simulink model "Automotive_Wiper"  (R2022b)
settings: Solver=FixedStepAuto  StartTime=0.0  StopTime=16  FixedStep=0.01  RelTol=1e-3
model workspace (MAT data in the model file):
  lowPathFilterGain = Simulink.Parameter
  lowPathFilterGain.Value = 0.1
  lowPathFilterGain.DataType = 'double'
  lowPathFilterGain.Complexity = 'real'
  lowPathFilterGain.Dimensions = [1 1]
undefined symbols (not defined in the file or in its folder): sigbuilder_block
libraries: simulink x1
settings Model: NumberOfSteps=100  VariantFading=off  Creator=mohsa  LastModifiedBy=mohsa
settings OptimizationCC: DefaultParameterBehavior=Inlined  UseDivisionForNetSlopeComputation=on  GainParamInheritBuiltInType=on  UseFloatMulNetSlope=on  InlineInvariantSignals=on  PassReuseOutputArgsAs=Individual arguments  ZeroExternalMemoryAtStartup=off  ZeroInternalMemoryAtStartup=off  NoFixptDivByZeroProtection=on  EfficientFloat2IntCast=on  LifeSpan=1  OptimizeBlockOrder=speed  DifferentSizesBufferReuse=on  EfficientTunableParamExpr=on
settings DebuggingCC: ParameterPrecisionLossMsg=none  ParameterTunabilityLossMsg=error
settings HardwareCC: ProdBitPerPointer=32  ProdBitPerSizeT=32  ProdBitPerPtrDiffT=32  ProdLargestAtomicInteger=Long  ProdLargestAtomicFloat=Double  ProdWordSize=32  ProdLongLongMode=on  ProdHWDeviceType=ARM Compatible->ARM Cortex-M
settings SFSimCC: MATLABDynamicMemAlloc=off
settings RTWCC: Description=Embedded Coder  SystemTargetFile=ert.tlc  TemplateMakefile=ert_default_tmf
settings CodeAppCC: ForceParamTrailComments=on  IgnoreCustomStorageClasses=off  OperatorAnnotations=on  SimulinkDataObjDesc=on  SFDataObjDesc=on  CustomSymbolStrGlobalVar=rt$N$M  CustomSymbolStrType=$N$M  CustomSymbolStrFcn=$N$M$F  CustomSymbolStrMacro=$N$M  InsertBlockDesc=on
settings ERTTargetCC: TargetLangStandard=C99 (ISO)  GenerateSampleERTMain=on  IncludeMdlTerminateFcn=off  CombineSignalStateStructs=on  SupportComplex=off  SupportNonInlinedSFcns=on  InlinedParameterPlacement=NonHierarchical  ERTCustomFileTemplate=example_file_process.tlc  ERTFilePackagingFormat=CompactWithDataFile

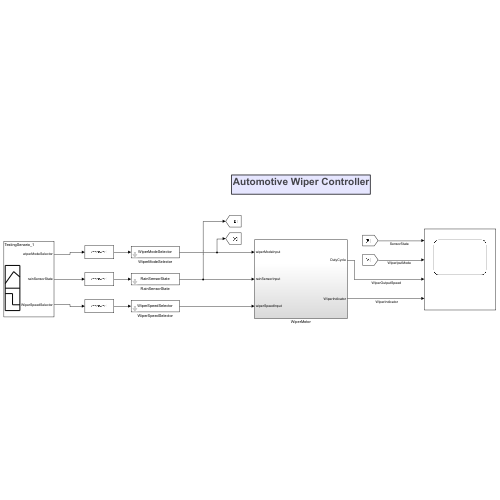
[thumbnail: Simulink's stored preview of the top-level diagram]
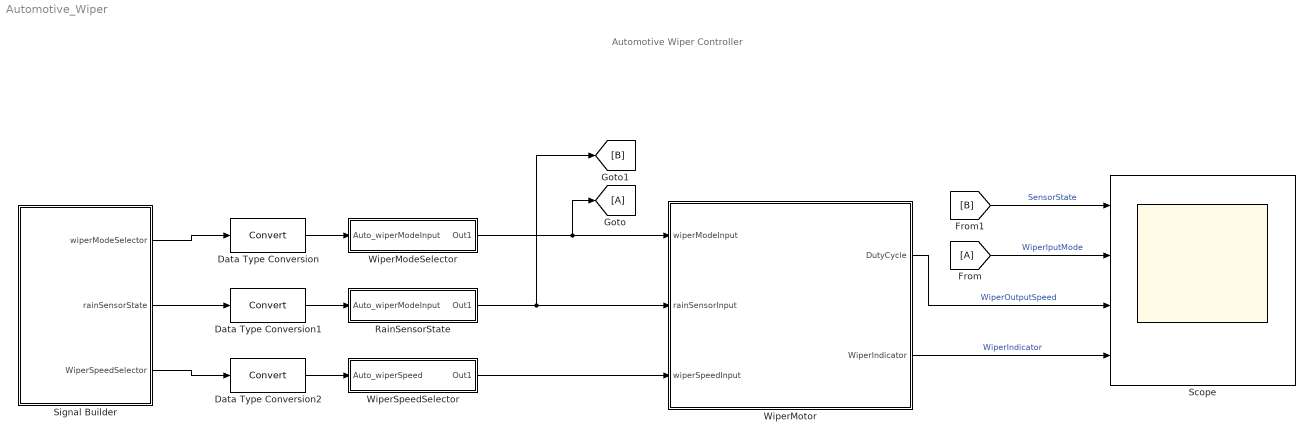
== system Automotive_Wiper ==
  note: Automotive Wiper Controller
  Data Type Conversion : DataTypeConversion  SaturateOnIntegerOverflow=off  RndMeth=Floor
  Data Type Conversion1 : DataTypeConversion  SaturateOnIntegerOverflow=off  RndMeth=Floor
  Data Type Conversion2 : DataTypeConversion  SaturateOnIntegerOverflow=off  RndMeth=Floor
  From : From
  Goto : Goto
  RainSensorState : Subsystem  mask{DebugMode=(1) Automatic debugging mode via InPort, rainSensorState=0}
      mask prompts: DebugMode "Debug Mode"; rainSensorState "Select State"
      mask TypeOptions DebugMode: (1) Automatic debugging mode via InPort | (2) Manual debugging mode via user input "Select State" below
      mask DialogControl s Prompt: %<MaskType> Rain Sensor Status
      mask DialogControl DescTextVar Prompt: %<MaskDescription>Set rain sensor status
      mask DialogControl Control2 Prompt: 0 = Normal
      mask DialogControl Control2_copy Prompt: 1 = Error
      mask Display: disp('RainSensorState');
  Scope : Scope  NumInputPorts=4
  Signal Builder : Subsystem  Tag=STV Subsys  LoadFcn=sigbuilder_block('load');  StartFcn=sigbuilder_block('start');  StopFcn=sigbuilder_block('stop');  ClipboardFcn=sigbuilder_block('clipboard');  mask(Sigbuilder block){tuvar=[0:10]}
      mask help: Simulink:masks:SigbuilderBlock_MD
      mask init:
      | if ~strcmp(get_param(bdroot(gcbh),'SimulationStatus'),'stopped') tuvar = sigbuilder_block('maskInit'); end
      settings: CopyFcn=sigbuilder_block('copy');  DeleteFcn=sigbuilder_block('delete');  ModelCloseFcn=sigbuilder_block('modelClose');  PreSaveFcn=sigbuilder_block('preSave');  PauseFcn=sigbuilder_block('pause');  ContinueFcn=sigbuilder_block('continue');  NameChangeFcn=sigbuilder_block('namechange');  OpenFcn=sigbuilder_block('open',[889.5 261 544.5 318.75 ]);  CloseFcn=sigbuilder_block('close');
      mask Display: plot(0, 0, 100, 100,[2, 2, 32, 32, 2], [68, 8, 8, 68, 68],[32, 2], [38, 38], [32, 19, 2],[53, 60, 44], [32, 17, 17, 2],[16, 16, 31, 31]);txt = getActiveGroup(gcbh);text(2, 100, txt,'verticalAlignment', 'top');
  WiperModeSelector : Subsystem  mask{DebugMode=(1) Automatic debugging mode via InPort, wiperModeInput=0}
      mask prompts: DebugMode "Debug Mode"; wiperModeInput "Select Mode"
      mask TypeOptions DebugMode: (1) Automatic debugging mode via InPort | (2) Manual debugging mode via user input "Select Mode" below
      mask DialogControl s Prompt: %<MaskType> Wiper Mode Selector
      mask DialogControl DescTextVar Prompt: %<MaskDescription>Select Wiper Operation mode
      mask DialogControl Control2 Prompt: 0 = OFF
      mask DialogControl Control2_copy Prompt: 1 = Auto Mode (Select Speed)
      mask DialogControl Control2_copy_copy Prompt: 2 = Low Speed Mode (40%)
      mask DialogControl Control2_copy_copy_copy Prompt: 3 = High Speed Mode (70%)
      mask Display: disp('WiperModeSelector');
  WiperMotor : Subsystem
  WiperSpeedSelector : Subsystem  mask{DebugMode=(1) Automatic debugging mode via InPort, wiperSpeed=0}
      mask prompts: DebugMode "Debug Mode"; wiperSpeed "Select Speed"
      mask TypeOptions DebugMode: (1) Automatic debugging mode via InPort | (2) Manual debugging mode via user input "Select Speed" below
      mask DialogControl s Prompt: %<MaskType> Rain Sensor Status
      mask DialogControl DescTextVar Prompt: %<MaskDescription>Set rain sensor status
      mask DialogControl Control0 Prompt: 0 = OFF
      mask DialogControl Control1 Prompt: 1 = 40% DutyCycle
      mask DialogControl Control2 Prompt: 2 = 45% DutyCycle
      mask DialogControl Control3 Prompt: 3 = 50% Duty Cycle
      mask DialogControl Control4 Prompt: 4 = 55% Duty Cycle
      mask DialogControl Control5 Prompt: 5 = 60% Duty Cycle
      mask DialogControl Control6 Prompt: 6 = 65% Duty Cycle
      mask DialogControl Control7 Prompt: 7 = 70% Duty Cycle
      mask Display: disp('WiperSpeedSelector');
  wires:
  Signal Builder/1(wiperModeSelector) -> Data Type Conversion/1
  Signal Builder/2(rainSensorState) -> Data Type Conversion1/1
  Signal Builder/3(WiperSpeedSelector) -> Data Type Conversion2/1
  Data Type Conversion/1 -> WiperModeSelector/1(Auto_wiperModeInput)
  Data Type Conversion1/1 -> RainSensorState/1(Auto_wiperModeInput)
  Data Type Conversion2/1 -> WiperSpeedSelector/1(Auto_wiperSpeed)
  WiperModeSelector/1(Out1) -> Goto/1, WiperMotor/1(wiperModeInput)
  RainSensorState/1(Out1) -> [B], WiperMotor/2(rainSensorInput)
  WiperSpeedSelector/1(Out1) -> WiperMotor/3(wiperSpeedInput)
  WiperMotor/1(DutyCycle) -> Scope/3  "WiperOutputSpeed"
  WiperMotor/2(WiperIndicator) -> Scope/4  "WiperIndicator"
  From/1 -> Scope/2  "WiperIputMode"
  [B] -> Scope/1  "SensorState"

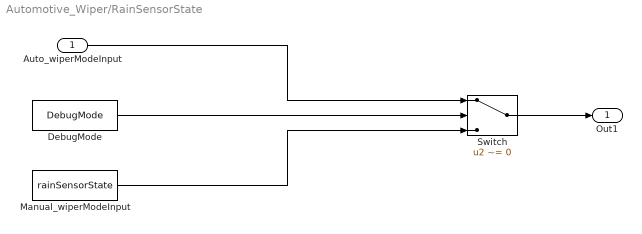
== system Automotive_Wiper/RainSensorState ==
  Auto_wiperModeInput : Inport
  DebugMode : Constant  Value=DebugMode
  Manual_wiperModeInput : Constant  Value=rainSensorState
  Switch : Switch  Criteria=u2 ~= 0  SaturateOnIntegerOverflow=off  InputSameDT=off
  Out1 : Outport
  wires:
  Auto_wiperModeInput/1 -> Switch/1
  Manual_wiperModeInput/1 -> Switch/3
  Switch/1 -> Out1/1
  DebugMode/1 -> Switch/2

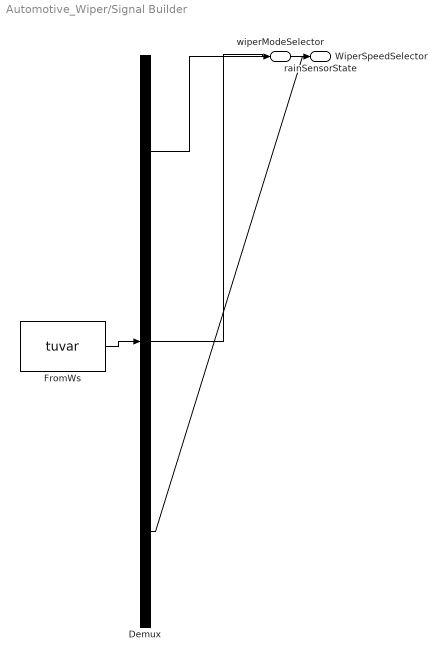
== system Automotive_Wiper/Signal Builder ==
  Demux : Demux  Tag=STV Demux  Outputs=3
      settings: DisplayOption=none
  FromWs : FromWorkspace  Tag=STV FromWs  VariableName=tuvar  SampleTime=1  OutputAfterFinalValue=Holding final value
      SigBuilderData=|
      | common.afterFinalStr = 'Hold final value'
      | common.sampleTime = '1'
      | dataSet.timeRange = [0 16]
      | dataSet.name = 'TestingSenario_1'
      | sbobj.Groups.Name = 'TestingSenario_1'
      | sbobj.Groups.Signals(1).Name = 'wiperModeSelector'
      | sbobj.Groups.Signals(1).XData = [0 1 2 3 4 5 6 7 8 9 10 11 12 13 14 15 16]
      | sbobj.Groups.Signals(1).YData = [0 0 2 2 3 3 1 1 1 1 1 1 1 1 1 1 1]
      | sbobj.Groups.Signals(2).Name = 'rainSensorState'
      | sbobj.Groups.Signals(2).XData = [0 1 2 3 4 5 6 7 8 9 10 11 12 13 14 15 16]
      | sbobj.Groups.Signals(2).YData = [0 0 0 0 0 0 0 0 0 0 0 0 0 0 0 1 0]
      | sbobj.Groups.Signals(3).Name = 'WiperSpeedSelector'
      | sbobj.Groups.Signals(3).XData = [0 1 2 3 4 5 6 7 8 9 10 11 12 13 14 15 16]
      | sbobj.Groups.Signals(3).YData = [0 0 0 0 0 0 0 0 1 2 3 4 5 6 7 7 7]
      | sbobj.Groups.TimeRange = [0 16]
  wiperModeSelector : Outport  Tag=STV Outport
  rainSensorState : Outport  Tag=STV Outport  Port=2
  WiperSpeedSelector : Outport  Tag=STV Outport  Port=3
  wires:
  Demux/1 -> wiperModeSelector/1
  FromWs/1 -> Demux/1
  Demux/2 -> rainSensorState/1
  Demux/3 -> WiperSpeedSelector/1

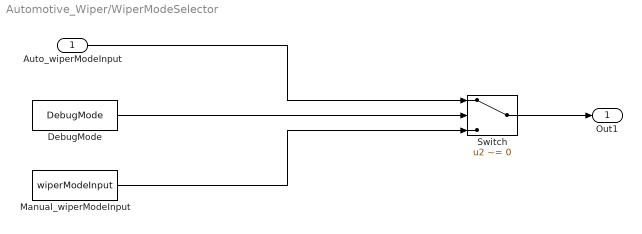
== system Automotive_Wiper/WiperModeSelector ==
  Auto_wiperModeInput : Inport
  DebugMode : Constant  Value=DebugMode  OutDataTypeStr=uint8
  Manual_wiperModeInput : Constant  Value=wiperModeInput  OutDataTypeStr=uint8
  Switch : Switch  Criteria=u2 ~= 0  SaturateOnIntegerOverflow=off  InputSameDT=off
  Out1 : Outport
  wires:
  Auto_wiperModeInput/1 -> Switch/1
  Manual_wiperModeInput/1 -> Switch/3
  Switch/1 -> Out1/1
  DebugMode/1 -> Switch/2

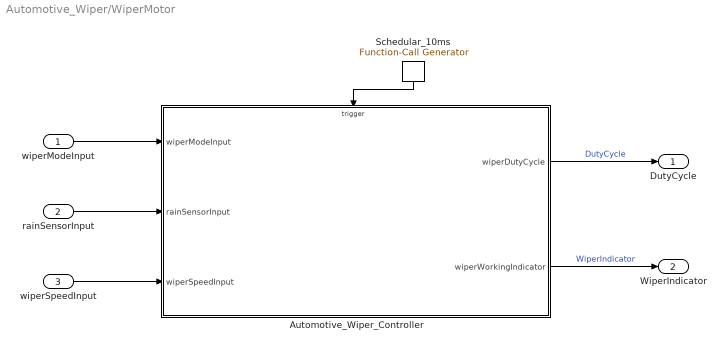
== system Automotive_Wiper/WiperMotor ==
  wiperModeInput : Inport
  rainSensorInput : Inport  Port=2
  wiperSpeedInput : Inport  Port=3
  Automotive_Wiper_Controller : Subsystem  TreatAsAtomicUnit=on
  Schedular_10ms : simulink/Ports & Subsystems/Function-Call Generator  sample_time=0  numberOfIterations=1  DisallowWideOutput=off
  DutyCycle : Outport
  WiperIndicator : Outport  Port=2
  wires:
  Automotive_Wiper_Controller/2(wiperWorkingIndicator) -> WiperIndicator/1  "WiperIndicator"
  Schedular_10ms/1 -> Automotive_Wiper_Controller/Trigger
  Automotive_Wiper_Controller/1(wiperDutyCycle) -> DutyCycle/1  "DutyCycle"
  wiperSpeedInput/1 -> Automotive_Wiper_Controller/3(wiperSpeedInput)
  wiperModeInput/1 -> Automotive_Wiper_Controller/1(wiperModeInput)
  rainSensorInput/1 -> Automotive_Wiper_Controller/2(rainSensorInput)

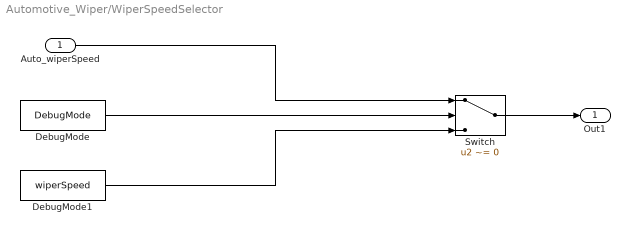
== system Automotive_Wiper/WiperSpeedSelector ==
  Auto_wiperSpeed : Inport
  DebugMode : Constant  Value=DebugMode  OutDataTypeStr=uint8
  DebugMode1 : Constant  Value=wiperSpeed  OutDataTypeStr=uint8
  Switch : Switch  Criteria=u2 ~= 0  SaturateOnIntegerOverflow=off  InputSameDT=off
  Out1 : Outport
  wires:
  Auto_wiperSpeed/1 -> Switch/1
  DebugMode1/1 -> Switch/3
  Switch/1 -> Out1/1
  DebugMode/1 -> Switch/2

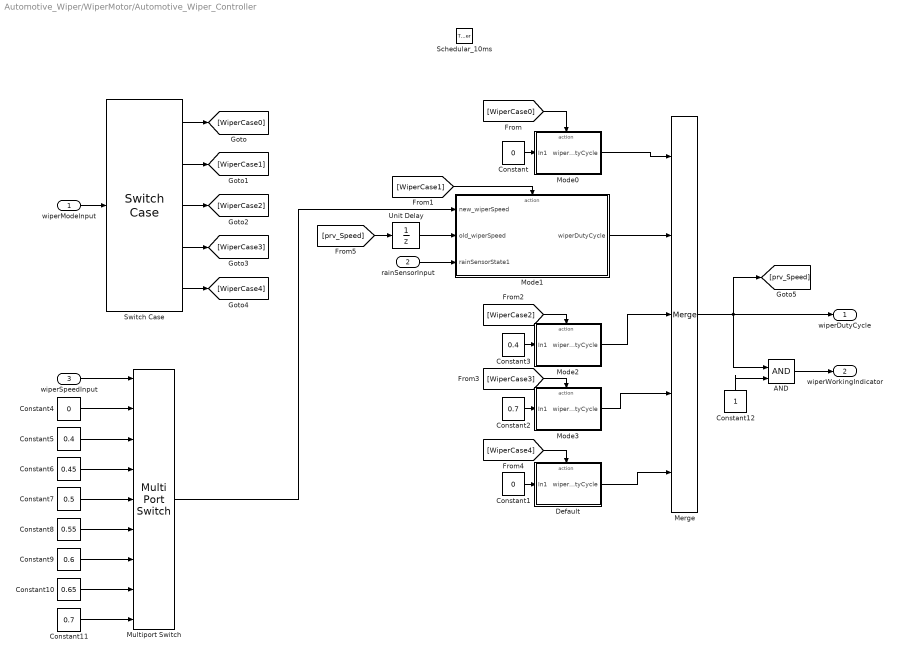
== system Automotive_Wiper/WiperMotor/Automotive_Wiper_Controller ==
  wiperModeInput : Inport
  rainSensorInput : Inport  Port=2
  wiperSpeedInput : Inport  Port=3
  Schedular_10ms : TriggerPort  TriggerType=function-call  VariantControl=(inherit)
  AND : Logic  IconShape=distinctive  AllPortsSameDT=off  OutDataTypeStr=boolean
  Constant : Constant  Value=0  OutDataTypeStr=double
  Constant1 : Constant  Value=0  OutDataTypeStr=double
  Constant10 : Constant  Value=0.65  OutDataTypeStr=double
  Constant11 : Constant  Value=0.7  OutDataTypeStr=double
  Constant12 : Constant
  Constant2 : Constant  Value=0.7  OutDataTypeStr=double
  Constant3 : Constant  Value=0.4  OutDataTypeStr=double
  Constant4 : Constant  Value=0  OutDataTypeStr=double
  Constant5 : Constant  Value=0.4  OutDataTypeStr=double
  Constant6 : Constant  Value=0.45  OutDataTypeStr=double
  Constant7 : Constant  Value=0.5  OutDataTypeStr=double
  Constant8 : Constant  Value=0.55  OutDataTypeStr=double
  Constant9 : Constant  Value=0.6  OutDataTypeStr=double
  Default : Subsystem  TreatAsAtomicUnit=on
  Merge : Merge  Inputs=5
  Mode0 : Subsystem  TreatAsAtomicUnit=on
  Mode1 : Subsystem  TreatAsAtomicUnit=on
  Mode2 : Subsystem  TreatAsAtomicUnit=on
  Mode3 : Subsystem  TreatAsAtomicUnit=on
  Multiport Switch : MultiPortSwitch  DataPortOrder=Zero-based contiguous  Inputs=8  zeroidx=on  SaturateOnIntegerOverflow=off  InputSameDT=off
  Switch Case : SwitchCase  CaseConditions={0 1 2 3}
  Unit Delay : UnitDelay  SampleTime=-1  HasFrameUpgradeWarning=on
  wiperDutyCycle : Outport
  wiperWorkingIndicator : Outport  Port=2
  wires:
  wiperModeInput/1 -> Switch Case/1
  Constant/1 -> Mode0/1(In1)
  Mode0/1(wiperDutyCycle) -> Merge/1
  Mode1/1(wiperDutyCycle) -> Merge/2
  Mode2/1(wiperDutyCycle) -> Merge/3
  Mode3/1(wiperDutyCycle) -> Merge/4
  Default/1(wiperDutyCycle) -> Merge/5
  [WiperCase0] -> Mode0/Action
  Switch Case/1 -> [WiperCase0]
  [WiperCase1] -> Mode1/Action
  [WiperCase2] -> Mode2/Action
  [WiperCase3] -> Mode3/Action
  [WiperCase4] -> Default/Action
  Switch Case/2 -> [WiperCase1]
  Switch Case/3 -> [WiperCase2]
  Switch Case/4 -> [WiperCase3]
  Switch Case/5 -> [WiperCase4]
  Constant1/1 -> Default/1(In1)
  Constant2/1 -> Mode3/1(In1)
  Constant3/1 -> Mode2/1(In1)
  Merge/1 -> [prv_Speed], AND/1, wiperDutyCycle/1
  rainSensorInput/1 -> Mode1/3(rainSensorState1)
  wiperSpeedInput/1 -> Multiport Switch/1
  Constant4/1 -> Multiport Switch/2
  Constant5/1 -> Multiport Switch/3
  Constant6/1 -> Multiport Switch/4
  Constant7/1 -> Multiport Switch/5
  Constant8/1 -> Multiport Switch/6
  Constant9/1 -> Multiport Switch/7
  Constant10/1 -> Multiport Switch/8
  Constant11/1 -> Multiport Switch/9
  Multiport Switch/1 -> Mode1/1(new_wiperSpeed)
  Unit Delay/1 -> Mode1/2(old_wiperSpeed)
  [prv_Speed] -> Unit Delay/1
  Constant12/1 -> AND/2
  AND/1 -> wiperWorkingIndicator/1

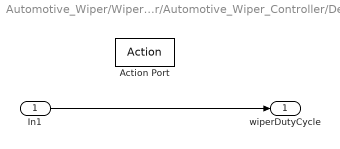
== system Automotive_Wiper/WiperMotor/Automotive_Wiper_Controller/Default ==
  In1 : Inport
  Action Port : ActionPort  ActionPortLabel=default:
  wiperDutyCycle : Outport
  wires:
  In1/1 -> wiperDutyCycle/1

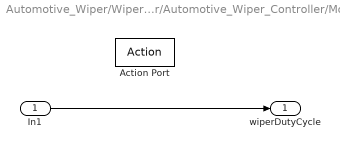
== system Automotive_Wiper/WiperMotor/Automotive_Wiper_Controller/Mode0 ==
  In1 : Inport
  Action Port : ActionPort  ActionPortLabel=case [ 0 ]:
  wiperDutyCycle : Outport
  wires:
  In1/1 -> wiperDutyCycle/1

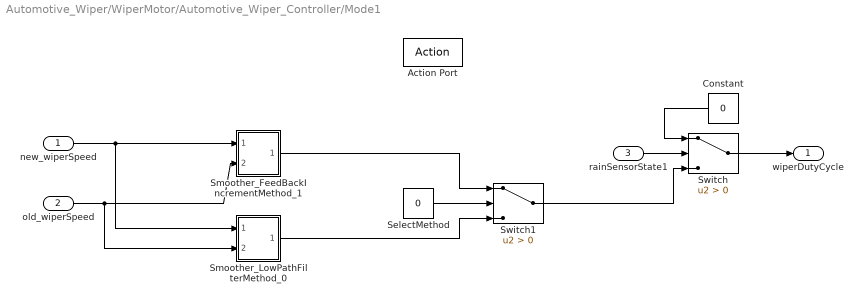
== system Automotive_Wiper/WiperMotor/Automotive_Wiper_Controller/Mode1 ==
  new_wiperSpeed : Inport  OutDataTypeStr=double
  old_wiperSpeed : Inport  Port=2  OutDataTypeStr=double
  rainSensorState1 : Inport  Port=3  OutDataTypeStr=uint8
  Action Port : ActionPort  ActionPortLabel=case [ 1 ]:
  Constant : Constant  Value=0  OutDataTypeStr=uint8
  SelectMethod : Constant  Value=0  OutDataTypeStr=uint8
  Smoother_FeedBackIncrementMethod_1 : Subsystem
  Smoother_LowPathFilterMethod_0 : Subsystem
  Switch : Switch  Criteria=u2 > Threshold  SaturateOnIntegerOverflow=off  InputSameDT=off
  Switch1 : Switch  Criteria=u2 > Threshold  SaturateOnIntegerOverflow=off  InputSameDT=off
  wiperDutyCycle : Outport
  wires:
  new_wiperSpeed/1 -> Smoother_LowPathFilterMethod_0/1(In1), Smoother_FeedBackIncrementMethod_1/1(In1)
  old_wiperSpeed/1 -> Smoother_FeedBackIncrementMethod_1/2(In2), Smoother_LowPathFilterMethod_0/2(In2)
  rainSensorState1/1 -> Switch/2
  Switch/1 -> wiperDutyCycle/1
  Constant/1 -> Switch/1
  Smoother_FeedBackIncrementMethod_1/1(Out1) -> Switch1/1
  Smoother_LowPathFilterMethod_0/1(Out1) -> Switch1/3
  SelectMethod/1 -> Switch1/2
  Switch1/1 -> Switch/3

== system Automotive_Wiper/WiperMotor/Automotive_Wiper_Controller/Mode2 ==
  In1 : Inport
  Action Port : ActionPort  ActionPortLabel=case [ 2 ]:
  wiperDutyCycle : Outport
  wires:
  In1/1 -> wiperDutyCycle/1

== system Automotive_Wiper/WiperMotor/Automotive_Wiper_Controller/Mode3 ==
  In1 : Inport
  Action Port : ActionPort  ActionPortLabel=case [ 3 ]:
  wiperDutyCycle : Outport
  wires:
  In1/1 -> wiperDutyCycle/1

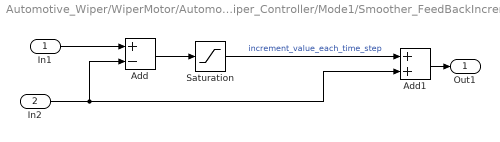
== system Automotive_Wiper/WiperMotor/Automotive_Wiper_Controller/Mode1/Smoother_FeedBackIncrementMethod_1 ==
  In1 : Inport
  In2 : Inport  Port=2
  Add : Sum  Inputs=+-
  Add1 : Sum
  Saturation : Saturate  UpperLimit=0.01  LowerLimit=-0.01
  Out1 : Outport
  wires:
  Add/1 -> Saturation/1
  Saturation/1 -> Add1/1  "increment_value_each_time_step"
  In1/1 -> Add/1
  In2/1 -> Add/2, Add1/2
  Add1/1 -> Out1/1

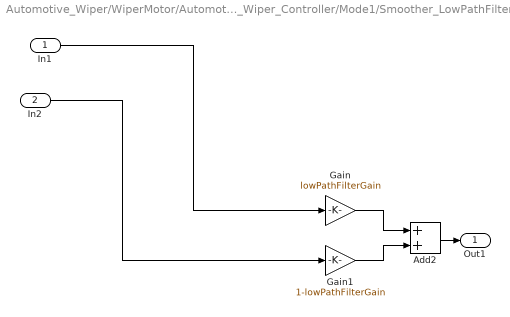
== system Automotive_Wiper/WiperMotor/Automotive_Wiper_Controller/Mode1/Smoother_LowPathFilterMethod_0 ==
  In1 : Inport
  In2 : Inport  Port=2
  Add2 : Sum
  Gain : Gain  Gain=lowPathFilterGain
  Gain1 : Gain  Gain=1-lowPathFilterGain
  Out1 : Outport
  wires:
  Gain1/1 -> Add2/2
  Add2/1 -> Out1/1
  In1/1 -> Gain/1
  In2/1 -> Gain1/1
  Gain/1 -> Add2/1
